simulink model "Microgrid_transition_model_092221"  (R2020a)
settings: Solver=VariableStepAuto  StartTime=0.0  StopTime=16  MaxStep=1e-4  RelTol=1e-3
PreLoadFcn:
  | %run('FC_microgrid_param.m')
  | %load('gen_grid_init.mat')
InitFcn:
  | %load myisoModel_init;
  | run('FC_microgrid_param.m')
  | tic
  | run('CARTinitFcn.m')
  | %caseNo = 2;
  | 
  | %if (caseNo == 1)
  | %set_param(['Isolated_grid_paper_model_022521/SignalGen'], 'ActiveScenario', 'PStep222kW');
  | %else
  | %set_param(['Isolated_grid_paper_model_022521/SignalGen'], 'ActiveScenario', 'QStep222kVAr');
  | 
  | %end;
StopFcn:
  | toc
undefined symbols (not defined in the file): breakpoints1, breakpoints2, cp_table_data, ctrl, D1, Delta, DiscIntNeverNeededParam, DT, FC_BESS, find_system, gcbh, libFC_BESS, LowerLimit, magnitude, oversize, pq_ts, sps_rtmsupport, timer, ts, Ts, Ts_APC, Ts_Control, Ts_Power, UpperLimit
libraries: powerlib x120, powerlib_meascontrol x85, simulink x63, powerlib_extras x40, simulink_extras x12, eePowerMeasurement x9, sps_avr x7, pi_ctrl x4, spsDieselMotorModel x3, SignalEditorBlockLib x2, libLgBattery x1, libFC_PV x1
(part 3 of 11)

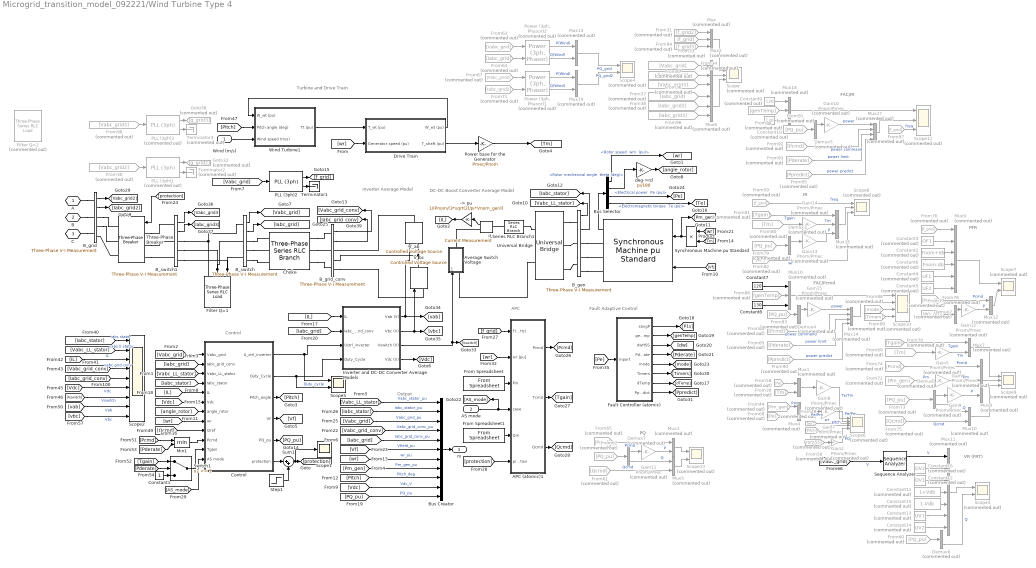
== system Microgrid_transition_model_092221/Wind Turbine Type 4 ==
  note: Control
  note: Turbine and Drive Train
  note: Inverter
      | Average Model
  note: DC-DC Boost Converter
      | Average Model
  note: Fault Adaptive Control
  note: PFR
  note: IR
  note: FAC/Pcmd
  note: PQ
  note: FAC/IR
  note: APC
  note: Output
  note: VR (FRT)
  "Wind (m/s) " : Inport
  AS mode : Inport  Port=2
  -> pu : Gain  Gain=1/(Pnom/(3*sqrt(2)/pi*Vnom_gen))  SaturateOnIntegerOverflow=on  OutDataTypeStr=Inherit: Same as input  ParamDataTypeStr=Inherit: Same as input
  APC (atomic)1 : Subsystem  TreatAsAtomicUnit=on  SystemSampleTime=0.01
  Average Switch Voltage : Subsystem
  B_gen : powerlib/Measurements/Three-Phase V-I Measurement  VoltageMeasurement=phase-to-phase  SetLabelV=off  LabelV=Vabc  Vpu=on  VpuLL=off  CurrentMeasurement=yes  SetLabelI=off  LabelI=Iabc  Ipu=on  Pbase=Pnom  Vbase=Vnom_gen  OutputType=Complex  PhasorSimulation=off  PSBequivalent=0
      settings: SourceProductBaseCode=MT,PS
  B_grid : powerlib/Measurements/Three-Phase V-I Measurement  VoltageMeasurement=phase-to-ground  SetLabelV=off  LabelV=Vabc  Vpu=off  VpuLL=off  CurrentMeasurement=yes  SetLabelI=off  LabelI=Iabc  Ipu=off  Pbase=Pnom  Vbase=Vnom  OutputType=Complex  PhasorSimulation=off  PSBequivalent=0
      settings: SourceProductBaseCode=MT,PS
  B_grid_conv : powerlib/Measurements/Three-Phase V-I Measurement  VoltageMeasurement=phase-to-ground  SetLabelV=off  LabelV=Vabc  Vpu=on  VpuLL=off  CurrentMeasurement=yes  SetLabelI=off  LabelI=Iabc  Ipu=on  Pbase=Pnom  Vbase=Vnom  OutputType=Complex  PhasorSimulation=off  PSBequivalent=0
      settings: SourceProductBaseCode=MT,PS
  B_switch : powerlib/Measurements/Three-Phase V-I Measurement  VoltageMeasurement=phase-to-ground  SetLabelV=off  LabelV=Vabc  Vpu=on  VpuLL=off  CurrentMeasurement=yes  SetLabelI=off  LabelI=Iabc  Ipu=on  Pbase=Pnom  Vbase=Vnom  OutputType=Complex  PhasorSimulation=off  PSBequivalent=0
      settings: SourceProductBaseCode=MT,PS
  B_switch1 : powerlib/Measurements/Three-Phase V-I Measurement  VoltageMeasurement=phase-to-ground  SetLabelV=off  LabelV=Vabc  Vpu=on  VpuLL=off  CurrentMeasurement=yes  SetLabelI=off  LabelI=Iabc  Ipu=on  Pbase=Pnom  Vbase=Vnom  OutputType=Complex  PhasorSimulation=off  PSBequivalent=0
      settings: SourceProductBaseCode=MT,PS
  Bus Creator : BusCreator  Inputs=11
  Bus Selector : BusSelector  OutputSignals="Mechanical.Rotor speed  wm  (pu),Mechanical.Rotor mechanical angle  theta (deg),Mechanical.Electrical power  Pe (pu),Mechanical.Electromagnetic torque  Te (pu)"
  "Choke " : powerlib/Elements/Three-Phase Series RLC Branch  LConnTagsString=A|B|C  RConnTagsString=A|B|C  BranchType=RL  Resistance=R_RL*Vnom^2/Pnom  Inductance=L_RL*Vnom^2/Pnom/(2*pi*Fnom)  Capacitance=[]  Measurements=None
      settings: SourceProductBaseCode=MT,PS
  Constant1 : Constant
  Constant10 : Constant  Commented=on  Value=130
  Constant11 : Constant  Commented=on  Value=1+Vdb
  Constant12 : Constant  Commented=on  Value=OV1
  Constant13 : Constant  Commented=on  Value=UV1
  Constant14 : Constant  Commented=on  Value=UV2
  Constant15 : Constant  Commented=on  Value=1-Vdb
  Constant16 : Constant  Commented=on  Value=OV2
  Constant2 : Constant  Commented=on  Value=Fnom+db
  Constant3 : Constant  Commented=on  Value=OF1
  Constant4 : Constant  Commented=on  Value=UF1
  Constant5 : Constant  Commented=on  Value=UF2
  Constant6 : Constant  Commented=on  Value=Fnom-db
  Constant7 : Constant  Value=120
  Constant8 : Constant  Value=130
  Constant9 : Constant  Commented=on  Value=120
  Control : Subsystem
  Demux{1..7} (7 alike) : Demux  Commented=on  Outputs=2
  Drive Train : Subsystem  mask(Wind Turbine shaft){H_WT=H_WT/10, Ksh=Ksh, D_mutual=D_mutual, wbase=2*pi*Fnom/p, w_wt0=w_wt0, torque0=torque0, Ts=Ts}
      mask prompts: H_WT "Wind turbine inertia constant H (s):"; Ksh "Shaft spring constant (pu of nominal mechanical torque/rad):"; D_mutual "Shaft mutual damping (pu of nominal mechanical torque/pu dw):"; wbase "Shaft base speed (rad/s):"; w_wt0 "Turbine initial speed (pu of base speed):"; torque0 "Initial output torque (pu of nominal mechanical torque):"; Ts "Sample time (s):"
      mask help:
      | This block implements a wind turbine drive train model. All shaft parameters are referred to high-speed shaft (generator shaft).
      |
      | The first input is the wind turbine torque in per unit (pu) based on the nominal power of the turbine and the base speed of the generator. The second input is the generator speed in pu based on the base speed of the generator.
      |
      | The outputs are:
      | 1- the transmitted torque of the shaft in pu based on the nominal power of the turbine and the base speed of the generator.
      | 2- the wind turbine speed in pu of the base speed of the generator.
  "Fault Controller (atomic) " : Subsystem  TreatAsAtomicUnit=on  SystemSampleTime=Ts_APC
  Filter Q=1 : powerlib/Elements/Three-Phase Series RLC Load  LConnTagsString=A|B|C  Configuration=Y (grounded)  NominalVoltage=Vnom  Vabc=[1e3 1e3 1e3]  Vabcp=[1e3 1e3 1e3]  NominalFrequency=Fnom  UnbalancedPower=off  ActivePower=100  InductivePower=100  CapacitivePower=100  Pabc=[10e3 9e3 11e3]  QLabc=[100 90 110]  QCabc=[100 90 110]  Pabcp=[10e3 9e3 11e3]  QLabcp=[100 90 110]  QCabcp=[100 90 110]  Measurements=None  LoadType=constant Z
      settings: SourceProductBaseCode=MT,PS
  Filter Q=2 : powerlib/Elements/Three-Phase Series RLC Load  Commented=on  LConnTagsString=A|B|C  Configuration=Y (grounded)  NominalVoltage=Vnom  Vabc=[1e3 1e3 1e3]  Vabcp=[1e3 1e3 1e3]  NominalFrequency=Fnom  UnbalancedPower=off  ActivePower=C_var_filter/Q_filter  InductivePower=0  CapacitivePower=C_var_filter  Pabc=[10e3 9e3 11e3]  QLabc=[100 90 110]  QCabc=[100 90 110]  Pabcp=[10e3 9e3 11e3]  QLabcp=[100 90 110]  QCabcp=[100 90 110]  Measurements=None  LoadType=constant Z
      settings: SourceProductBaseCode=MT,PS
  From Spreadsheet : FromSpreadsheet  FileName=Microgrid_cmd.xlsx  SheetName=P  SampleTime=Ts_APC
  From Spreadsheet1 : FromSpreadsheet  FileName=Microgrid_cmd.xlsx  SheetName=Q  SampleTime=Ts_APC
  From30 : From  Commented=on  GotoTag=Vabc_grid2
  From31 : From  Commented=on  GotoTag=f_grid2
  From{33,59,76,97} (4 alike) : From  Commented=on  GotoTag=f_grid
  From34 : From  Commented=on  GotoTag=Vabc_grid
  From36 : From  Commented=on  GotoTag=Vabc_grid2
  From37 : From  Commented=on  GotoTag=Iabc_grid
  From38 : From  Commented=on  GotoTag=Iabc_grid2
  From39 : From  Commented=on  GotoTag=Tm
  From44 : From  Commented=on  GotoTag=Pm_gen
  From48 : From  Commented=on  GotoTag=wr
  From55 : From  Commented=on  GotoTag=Pitch
  From{56,60,62,73,77,79,83,91} (8 alike) : From  Commented=on  GotoTag=PQ_pu
  From58 : From  Commented=on  GotoTag=Te
  From61 : From  Commented=on  GotoTag=Qcmd
  From63 : From  Commented=on  GotoTag=Vabc_grid
  From64 : From  Commented=on  GotoTag=Iabc_grid
  From{65,74,78,84,92} (5 alike) : From  Commented=on  GotoTag=Pcmd
  From67 : From  Commented=on  GotoTag=Vabc_grid2
  From68 : From  Commented=on  GotoTag=Pe
  From69 : From  Commented=on  GotoTag=Tm
  From70 : From  Commented=on  GotoTag=Tgain
  From71 : From  Commented=on  GotoTag=Iabc_grid2
  From72 : From  Commented=on  GotoTag=Pm_gen
  From75 : From  Commented=on  GotoTag=Qcmd
  From80 : From  Commented=on  GotoTag=Tm
  From81 : From  Commented=on  GotoTag=Tgain
  From82 : From  Commented=on  GotoTag=wr
  From85 : From  Commented=on  GotoTag=Pderate
  From86 : From  Commented=on  GotoTag=genTemp
  From87 : From  Commented=on  GotoTag=Vabc_grid3
  From88 : From  Commented=on  GotoTag=mode
  From89 : From  Commented=on  GotoTag=Timers
  From90 : From  Commented=on  GotoTag=Ppredict
  From93 : From  Commented=on  GotoTag=Pderate
  From94 : From  Commented=on  GotoTag=genTemp
  From95 : From  Commented=on  GotoTag=Ppredict
  From96 : From  Commented=on  GotoTag=Iabc_grid3
  From98 : From  Commented=on  GotoTag=Vabc_grid3
  From99 : From  Commented=on  GotoTag=f_grid3
  Gain{2,5..15} (12 alike) : Gain  Commented=on  Gain=Pnom/Pmec
  Goto32 : Goto  Commented=on  GotoTag=g_grid2
  Goto38 : Goto  Commented=on  GotoTag=g_grid3
  IL : powerlib/Measurements/Current Measurement  PhasorSimulation=off  OutputType=Complex  PSBequivalent=0
      settings: SourceProductBaseCode=MT,PS
  Inverter and DC-DC Converter Average Models : Subsystem
  Min1 : MinMax  Inputs=2
  Mux{,2,6,8,15..16,18} (7 alike) : Mux  Commented=on  Inputs=3
  Mux{1,3..5,7,10,12..13,19} (9 alike) : Mux  Commented=on  Inputs=2
  Mux11 : Mux  Commented=on  Inputs=7
  Mux14 : Mux  Commented=on
  Mux17 : Mux  Commented=on
  Mux9 : Mux  Commented=on  Inputs=6
  PLL (3ph)1 : powerlib_meascontrol/PLL/PLL (3ph)  Commented=on  Fmin=45  Par_Init=[0, 60]  ParK=[180, 3200, 1]  TcD=1e-4  MaxRateChangeFreq=12  FilterCutOffFreq=25  Ts=Ts  AGC=on
  PLL (3ph)2 : powerlib_meascontrol/PLL/PLL (3ph)  Fmin=45  Par_Init=[0, 60]  ParK=[180, 3200, 1]  TcD=1e-4  MaxRateChangeFreq=12  FilterCutOffFreq=25  Ts=Ts  AGC=on
  PLL (3ph)3 : powerlib_meascontrol/PLL/PLL (3ph)  Commented=on  Fmin=45  Par_Init=[0, 60]  ParK=[180, 3200, 1]  TcD=1e-4  MaxRateChangeFreq=12  FilterCutOffFreq=25  Ts=Ts  AGC=on
  "Power (3ph, Phasor)1" : powerlib_meascontrol/Measurements/Power (3ph, Phasor)  Commented=on
      settings: SourceProductBaseCode=PS
  "Power (3ph, Phasor)2" : powerlib_meascontrol/Measurements/Power (3ph, Phasor)  Commented=on
      settings: SourceProductBaseCode=PS
  Power base for the Generator : Gain  Gain=Pmec/Pnom  SaturateOnIntegerOverflow=on  OutDataTypeStr=Inherit: Same as input  ParamDataTypeStr=Inherit: Same as input
  Product : Product  RndMeth=Zero
  Scope{,8..9,11} (4 alike) : Scope  Commented=on  NumInputPorts=3
  Scope1 : Scope
  Scope10 : Scope  Commented=on  NumInputPorts=4
  Scope{3..4,7,13} (4 alike) : Scope  Commented=on  NumInputPorts=2
  Scope2 : Scope  NumInputPorts=9
  Scope5 : Scope  NumInputPorts=2
  Scope6 : Scope  Commented=on  NumInputPorts=5
  Sequence Analyzer : powerlib_meascontrol/Measurements/Sequence Analyzer  Freq=60  n=1  seq=Positive  InInit=[1, 0]  Ts=Ts
      settings: SourceProductBaseCode=PS
  Series RLC Branch1 : powerlib/Elements/Series RLC Branch  LConnTagsString=__new0  RConnTagsString=__new0  BranchType=RL  Resistance=R_Boost  Inductance=L_Boost  SetiL0=off  InitialCurrent=0  Capacitance=1.0  Setx0=off  InitialVoltage=0  Measurements=Branch current
      settings: SourceProductBaseCode=MT,PS
  Step1 : Step  Time=4  After=0  SampleTime=Ts
  Sum1 : Sum  Inputs=|++
  Switch1 : Switch  Threshold=1
  Synchronous Machine pu Standard : powerlib/Machines/Synchronous Machine pu Standard  PresetModel=No  MechanicalLoad=Mechanical power Pm  ShowDetailedParameters=on  RotorType=Salient-pole  Units=per unit standard parameters  MeasurementBus=off  NominalParameters="[ Pnom  Vnom_gen Fnom ]"  Reactances1=[ 1.81, 0.3, 0.23, 1.76, 0.65, 0.25, 0.15 ]  Reactances2="[ Xd, Xd1, Xd2, Xq,  Xq2,  Xl ]"  dAxisTimeConstants=Open-circuit  qAxisTimeConstants=Short-circuit  TimeConstants1="[ 4.4849  0.0681  0.1  ]"  TimeConstants2=[ 8.0, 0.03, 1.0, 0.07 ]  TimeConstants3="[  Tdo1  Tdo2  Tq2  ]"  TimeConstants4=[ 8.0, 0.03, 0.3371, 0.0295 ]  TimeConstants5=[ 1.01, 0.053, 0.1 ]  TimeConstants6=[ 1.3201, 0.023, 1.0, 0.07 ]  TimeConstants7="[  1.01  0.053  0.051266  ]"  TimeConstants8=[ 1.3201, 0.0231, 0.3371, 0.0295 ]  StatorResistance=Resistance  Mechanical=[ H F p]  PolePairs=1  InitialConditions=init  SetSaturation=off  Saturation=[0.6404,0.7127,0.8441,0.9214,0.9956,1.082,1.19,1.316,1.457;0.7,0.7698,0.8872,0.9466,0.9969,1.046,1.1,1.151,1.201]  LoadFlowParameters=[1,0,0,0,0]  TsPowergui=0  TsBlock=-1  IterativeModel=Trapezoidal non iterative  IterativeDiscreteModel=Trapezoidal non iterative  BusType=PV  Pref=0  Qref=0  Qmin=-inf  Qmax=inf  PLF=0  QLF=0
      settings: SourceProductBaseCode=MT,PS
  Terminator1 : Terminator
  Terminator2 : Terminator  Commented=on
  Terminator3 : Terminator  Commented=on
  Three-Phase Breaker : powerlib/Elements/Three-Phase Breaker  InitialState=closed  SwitchA=on  SwitchB=on  SwitchC=on  SwitchTimes=[1000]  External=on  BreakerResistance=Ron_breaker/Nb_WT  SnubberResistance=Rs_breaker/Nb_WT  SnubberCapacitance=Cs_breaker*Nb_WT  Measurements=None
  Universal Bridge : powerlib/Power Electronics/Universal Bridge  Arms=3  SnubberResistance=2*Ts_snub/(Pnom/(1000*2*pi*Fnom*Vnom_gen^2))  SnubberCapacitance=Pnom/(1000*2*pi*Fnom*Vnom_gen^2)  Device=Diodes  Ron=1e-6/Nb_wt  Lon=0  ForwardVoltages="[  0  0  ]"  ForwardVoltage=0  GTOparameters=[ 10e-6 , 20e-6 ]  IGBTparameters=[ 1e-6 , 2e-6 ]  Measurements=None  Measurements_2=None  converterType=Rectifier
      settings: SourceProductBaseCode=MT,PS
  V_ab : powerlib/Electrical Sources/Controlled Voltage Source  Initialize=on  Source_Type=AC  Amplitude=0  Phase=0  Frequency=0  Measurements=None
      settings: SourceProductBaseCode=MT,PS
  V_bc : powerlib/Electrical Sources/Controlled Voltage Source  Initialize=on  Source_Type=AC  Amplitude=0  Phase=0  Frequency=0  Measurements=None
      settings: SourceProductBaseCode=MT,PS
  Wind Turbine1 : Subsystem  mask(Wind Turbine){Prated=Pmec, c1_c8=c1_c8, K1_K2=K1_K2, wind0=wind0, Ts=Ts}
      mask prompts: Prated "Nominal mechanical output power (W):"; c1_c8 "Coefficients [c1 ... c8]"; K1_K2 "Parameters [K1 K2]"; wind0 "Initial wind speed (m/s):"; Ts "Sample time (s):"
      mask help:
      | This block implements a generic wind turbine models.
      |
      | The first input is the turbine speed in per unit of the generator base speed. For a synchronous or asynchronous generator, the base speed is the synchronous speed. For a permanent-magnet generator, the base speed is defined as the speed producing nominal voltage at  no load. The second input is the blade pitch angle in degrees. The third input is the wind speed in m/s.
      |
      | The output is the torque applied to the drive train in per unit based on the nominal power of the turbine and the base speed of the generator.
      mask init:
      | c1 = c1_c8(1);
      | c2 = c1_c8(2);
      | c3 = c1_c8(3);
      | c4 = c1_c8(4);
      | c5 = c1_c8(5);
      | c6 = c1_c8(6);
      | c7 = c1_c8(7);;
      | c8 = c1_c8(8);
      | 
      | K1=K1_K2(1);
      | K2=K1_K2(2);
      settings: OpenFcn=power_openblockproxy();
      mask Display: disp('');
  deg->rd : Gain  Gain=pi/180  SaturateOnIntegerOverflow=on  OutDataTypeStr=Inherit: Same as input  ParamDataTypeStr=Inherit: Same as input
  A : PMIOPort  Tag=PMCPort  Side=Left
  B : PMIOPort  Tag=PMCPort  Port=2  Side=Left
  C : PMIOPort  Tag=PMCPort  Port=3  Side=Left
  m : Outport  VectorParamsAs1DForOutWhenUnconnected=off
  wires:
  Bus Selector/2 -> deg->rd/1  "<Rotor mechanical angle  theta (deg)>"
  deg->rd/1 -> [angle_rotor]
  Bus Selector/1 -> [wr]  "<Rotor speed  wm  (pu)>"
  [Iabc_grid] -> Inverter and DC-DC Converter Average Models/2(Iabc_grid_conv)
  [IL] -> Inverter and DC-DC Converter Average Models/1(IL)
  [Vabc_grid] -> Control/1(Vabc_grid)
  [Iabc_grid] -> Control/2(Iabc_grid_conv)
  [Vabc_LL_stator] -> Control/3(Vabc_LL_stator)
  [Iabc_stator] -> Control/4(Iabc_stator)
  [Vdc] -> Control/6(Vdc)
  [angle_rotor] -> Control/7(angle_rotor)
  [wr] -> Control/8(wr)
  Control/2(Duty_Cycle) -> Scope5/2, Inverter and DC-DC Converter Average Models/4(Duty_Cycle)  "Duty_cycle"
  Control/3(Pitch_angle) -> [Pitch]
  Control/4(Vf) -> [Vf]
  Control/5(PQ_pu) -> [PQ_pu]
  [IL] -> Control/5(IL)
  Control/1(U_ctrl_inverter) -> Scope5/1, Inverter and DC-DC Converter Average Models/3(Uctrl_inverter)
  Inverter and DC-DC Converter Average Models/4(Vdc (V)) -> [Vdc]
  [Qcmd] -> Control/9(Qref)
  [Pitch] -> Wind Turbine1/2(Pitch angle (deg))
  Drive Train/2(T_shaft (pu)) -> Power base for the Generator/1
  Drive Train/1(W_wt (pu)) -> Wind Turbine1/1(W_wt (pu))
  "Wind (m/s) "/1 -> Wind Turbine1/3(Wind speed (m/s))
  Power base for the Generator/1 -> [Tm]
  [wr] -> Drive Train/2(Generator speed (pu))
  Wind Turbine1/1(Tt (pu)) -> Drive Train/1(T_wt (pu))
  Bus Selector/4 -> [Te]  "<Electromagnetic torque  Te (pu)>"
  Bus Selector/3 -> [Pe]  "<Electrical power  Pe (pu)>"
  Inverter and DC-DC Converter Average Models/1(Vab (V)) -> V_ab/1, [vab]
  [wr] -> Product/1
  B_gen/2 -> [Iabc_stator]
  Inverter and DC-DC Converter Average Models/2(Vbc (V)) -> V_bc/1, [vbc]
  B_switch/2 -> [Iabc_grid]
  Synchronous Machine pu Standard/1 -> Bus Selector/1
  B_switch/1 -> [Vabc_grid]
  [Tm] -> Product/2
  IL/1 -> -> pu/1
  B_gen/1 -> [Vabc_LL_stator]
  [Vf] -> Synchronous Machine pu Standard/2
  Inverter and DC-DC Converter Average Models/3(Vswitch (V)) -> Average Switch Voltage/1(Vswitch), [Vswitch]
  B_grid_conv/1 -> [Vabc_grid_conv]
  Product/1 -> Synchronous Machine pu Standard/1, [Pm_gen]
  -> pu/1 -> [IL]
  Control/6(protection) -> Sum1/1
  "Fault Controller (atomic) "/1(savgP) -> [P1s]
  [Pe] -> "Fault Controller (atomic) "/1(Inport)
  "Fault Controller (atomic) "/8(Ppredict) -> [Ppredict]
  "Fault Controller (atomic) "/2(genTemp) -> [genTemp]
  "Fault Controller (atomic) "/7(dTemp) -> [dTemp]
  "Fault Controller (atomic) "/6(Timers) -> [Timers]
  "Fault Controller (atomic) "/4(Pderate) -> [Pderate]
  "Fault Controller (atomic) "/3(dwHSS) -> [dw]
  "Fault Controller (atomic) "/5(mode) -> [mode]
  Gain8/1 -> Scope6/1  "Te/Tm"
  From80/1 -> Gain14/1
  From77/1 -> Demux2/1
  From39/1 -> Mux1/2
  Constant10/1 -> Mux18/3
  From75/1 -> Mux10/2  "Qcmd"
  Mux12/1 -> Scope7/2
  From74/1 -> Mux8/1  "Pcmd"
  From58/1 -> Mux1/1
  Mux9/1 -> Scope7/1
  From83/1 -> Demux4/1
  Gain13/1 -> Mux15/3  "P"
  Gain14/1 -> Mux15/2  "Tm"
  Gain12/1 -> Mux12/2  "P"
  From70/1 -> Mux7/1  "Tgain"
  Demux5/1 -> Gain10/1
  Gain9/1 -> Mux8/3  "P"
  From85/1 -> Mux14/3  "power limit"
  From68/1 -> Mux4/2
  From82/1 -> Scope8/3  "wr"
  Mux17/1 -> Scope11/2
  Demux1/1 -> Gain9/1
  From89/1 -> Scope10/4
  Mux5/1 -> Scope13/2
  Mux4/1 -> Gain7/1  "Pe/Pm"
  From59/1 -> Scope8/1  "freq"
  From90/1 -> Mux14/4  "power predict"
  Mux10/1 -> Scope9/3
  Demux1/2 -> Mux10/1  "Q"
  From44/1 -> Mux4/1  "Pm"
  From94/1 -> Mux18/2
  From55/1 -> Scope6/4  "pitch"
  Mux14/1 -> Scope10/2
  From56/1 -> Gain2/1
  Constant9/1 -> Mux18/1
  Constant8/1 -> Mux16/3
  From73/1 -> Demux1/1
  From93/1 -> Mux17/3  "power limit"
  From92/1 -> Mux17/2  "power command"
  Mux1/1 -> Gain8/1
  Mux8/1 -> Scope9/2
  Gain15/1 -> Mux14/1  "power"
  Constant2/1 -> Mux9/3
  Mux16/1 -> Scope10/1
  From84/1 -> Mux14/2  "power command"
  From78/1 -> Mux12/1  "Pcmd"
  Constant7/1 -> Mux16/1
  Mux15/1 -> Scope8/2
  From91/1 -> Demux5/1
  Gain11/1 -> Mux3/2  "P"
  Gain5/1 -> Mux7/2  "Tm"
  From72/1 -> Gain6/1  "Pm"
  From62/1 -> Demux7/1
  From97/1 -> Scope11/3  "freq"
  Gain10/1 -> Mux17/1  "power"
  From81/1 -> Mux15/1  "Tgain"
  Gain6/1 -> Mux8/2  "Pm"
  From61/1 -> Mux5/2  "Qcmd"
  From69/1 -> Gain5/1
  From48/1 -> Scope6/3  "wr"
  Mux3/1 -> Scope13/1
  Demux2/1 -> Gain12/1
  Demux4/1 -> Gain15/1
  Constant3/1 -> Mux9/2
  Constant5/1 -> Mux9/6
  Demux7/2 -> Mux5/1  "Q"
  From79/1 -> Demux3/1
  From65/1 -> Mux3/1  "Pcmd"
  From95/1 -> Mux17/4  "power predict"
  Constant6/1 -> Mux9/4
  Demux3/1 -> Gain13/1
  Constant4/1 -> Mux9/5
  Gain2/1 -> Scope6/5  "PQ"
  Demux7/1 -> Gain11/1
  Mux18/1 -> Scope11/1
  Mux7/1 -> Scope9/1
  From76/1 -> Mux9/1
  Gain7/1 -> Scope6/2  "Pe/Pm"
  From88/1 -> Scope10/3
  From86/1 -> Mux16/2
  [Pderate] -> Min1/2
  [Pcmd] -> Min1/1
  Min1/1 -> Control/10(Pcmd)
  [Pderate] -> Switch1/2
  Switch1/1 -> Control/11(Tgain)
  Constant1/1 -> Switch1/3
  [Tgain] -> Switch1/1
  PLL (3ph)2/2 -> Terminator1/1
  [Vabc_grid] -> PLL (3ph)2/1
  PLL (3ph)2/1 -> [f_grid]
  From Spreadsheet1/1 -> APC (atomic)1/5(Qin)
  [f_grid] -> APC (atomic)1/1(Freq (Hz))
  APC (atomic)1/3(Qcmd) -> [Qcmd]
  APC (atomic)1/2(Tcmd) -> [Tgain]
  [protection] -> APC (atomic)1/6(protection)
  [wr] -> APC (atomic)1/2(wr [pu])
  AS mode/1 -> APC (atomic)1/4(case), [AS_mode]
  APC (atomic)1/1(Pcmd) -> [Pcmd]
  From Spreadsheet/1 -> APC (atomic)1/3(Pin)
  [AS_mode] -> Control/12(AS mode)
  [Pm_gen] -> Bus Creator/8  "Pm_gen_pu"
  Bus Creator/1 -> m/1
  [Iabc_grid] -> Bus Creator/5  "Iabc_grid_conv_pu"
  [Pitch] -> Bus Creator/9  "Pitch_deg"
  [PQ_pu] -> Bus Creator/11  "PQ_pu"
  [Vf] -> Bus Creator/6  "Vfield_pu"
  [Vdc] -> Bus Creator/10  "Vdc_V"
  [Vabc_LL_stator] -> Bus Creator/1  "Vabc_stator_pu"
  [Vabc_grid] -> Bus Creator/3  "Vabc_grid_pu"
  [Iabc_stator] -> Bus Creator/2  "Iabc_stator_pu"
  [wr] -> Bus Creator/7  "wr_pu"
  [Vabc_grid_conv] -> Bus Creator/4  "Vabc_grid_conv_pu"
  B_grid/2 -> [Iabc_grid2]
  B_grid/1 -> [Vabc_grid2]
  PLL (3ph)1/1 -> Goto32/1
  PLL (3ph)1/2 -> Terminator2/1
  From30/1 -> PLL (3ph)1/1
  From31/1 -> Mux/1
  From33/1 -> Mux/2
  From34/1 -> Mux2/1
  From36/1 -> Mux2/2
  Mux2/1 -> Scope/2
  Mux/1 -> Scope/1
  [protection] -> Three-Phase Breaker/1
  Step1/1 -> Sum1/2
  Sum1/1 -> Scope1/1, [protection]
  [Iabc_stator] -> Scope2/1  "iabc stator"
  [Vabc_LL_stator] -> Scope2/2  "vabs ll stator"
  [IL] -> Scope2/3  "IL"
  [Vabc_grid_conv] -> Scope2/4  "vabc grid conv"
  [Vdc] -> Scope2/6  "Vdc"
  [Vswitch] -> Scope2/7  "Vswitch"
  [vab] -> Scope2/8  "Vab"
  [vbc] -> Scope2/9  "Vbc"
  Sequence Analyzer/1 -> Mux11/1  "V"
  Constant13/1 -> Mux11/6
  Constant15/1 -> Mux11/5
  Constant14/1 -> Mux11/7
  Constant12/1 -> Mux11/3
  Constant11/1 -> Mux11/4
  Mux11/1 -> Scope3/1
  [Vabc_grid] -> Sequence Analyzer/1  "V"
  Constant16/1 -> Mux11/2
  Demux6/2 -> Scope3/2  "Q"
  From60/1 -> Demux6/1
  "Power (3ph, Phasor)2"/2 -> Mux13/2  "Q(Wind)"
  From63/1 -> "Power (3ph, Phasor)2"/1
  "Power (3ph, Phasor)2"/1 -> Mux13/1  "P(Wind)"
  From64/1 -> "Power (3ph, Phasor)2"/2
  Mux13/1 -> Scope4/1  "PQ_grid"
  Mux19/1 -> Scope4/2  "PQ_grid2"
  From71/1 -> "Power (3ph, Phasor)1"/2
  From67/1 -> "Power (3ph, Phasor)1"/1
  "Power (3ph, Phasor)1"/1 -> Mux19/1  "P(Wind)"
  "Power (3ph, Phasor)1"/2 -> Mux19/2  "Q(Wind)"
  B_switch1/1 -> [Vabc_grid3]
  B_switch1/2 -> [Iabc_grid3]
  PLL (3ph)3/1 -> Goto38/1
  PLL (3ph)3/2 -> Terminator3/1
  From98/1 -> PLL (3ph)3/1
  From99/1 -> Mux/3
  From87/1 -> Mux2/3
  From37/1 -> Mux6/1
  From38/1 -> Mux6/2
  From96/1 -> Mux6/3
  Mux6/1 -> Scope/3
  B_grid_conv/2 -> [Iabc_grid_conv]
  [Iabc_grid_conv] -> Scope2/5
  connections:
  B_grid/RConn1 -- Three-Phase Breaker/RConn1
  B_grid/RConn2 -- Three-Phase Breaker/RConn2
  Three-Phase Breaker/RConn3 -- B_grid/RConn3
  B_grid_conv/RConn2 -- V_bc/RConn1 -- V_ab/LConn1
  Filter Q=1/LConn3 -- B_switch/LConn3 -- B_switch1/RConn3
  Filter Q=1/LConn2 -- B_switch/LConn2 -- B_switch1/RConn2
  B_switch/LConn1 -- B_switch1/RConn1 -- Filter Q=1/LConn1
  B_switch/RConn3 -- "Choke "/LConn3
  "Choke "/RConn3 -- B_grid_conv/LConn3
  B_switch/RConn2 -- "Choke "/LConn2
  Universal Bridge/LConn1 -- B_gen/LConn1
  B_gen/RConn2 -- Synchronous Machine pu Standard/RConn2
  Average Switch Voltage/RConn1 -- IL/RConn1
  Universal Bridge/LConn2 -- B_gen/LConn2
  Universal Bridge/LConn3 -- B_gen/LConn3
  V_ab/RConn1 -- B_grid_conv/RConn1
  B_switch/RConn1 -- "Choke "/LConn1
  B_gen/RConn1 -- Synchronous Machine pu Standard/RConn1
  "Choke "/RConn1 -- B_grid_conv/LConn1
  "Choke "/RConn2 -- B_grid_conv/LConn2
  B_grid_conv/RConn3 -- V_bc/LConn1
  Series RLC Branch1/LConn1 -- Universal Bridge/RConn1
  B_gen/RConn3 -- Synchronous Machine pu Standard/RConn3
  Series RLC Branch1/RConn1 -- IL/LConn1
  Average Switch Voltage/LConn1 -- Universal Bridge/RConn2
  A/RConn1 -- B_grid/LConn1
  B/RConn1 -- B_grid/LConn2
  C/RConn1 -- B_grid/LConn3
  Three-Phase Breaker/LConn1 -- B_switch1/LConn1
  Three-Phase Breaker/LConn2 -- B_switch1/LConn2
  Three-Phase Breaker/LConn3 -- B_switch1/LConn3

== system Microgrid_transition_model_092221/induction attempts2 ==
  Asynchronous Machine pu ABB 1.8MW : powerlib/Machines/Asynchronous Machine pu Units  Commented=on  RotorType=Squirrel-cage  PresetModel=No  MechanicalLoad=Torque Tm  ShowDetailedParameters=on  ReferenceFrame=Rotor  Units=pu  MeasurementBus=off  NominalParameters=[1.8e+06 1e+04 60]  Stator=[0.02565 0.09937]  Rotor=[0.01909 0.0397]  Cage1=[0.004672 0.11]  Cage2=[0.04455 0.09937]  Lm=3.275  Mechanical=[0.09526 0.05479 2]  PolePairs=2  InitialConditions="[ 0.01,0   0,0,0   0,0,0 ]"  SimulateSaturation=off  Saturation="[0.212,0.4201,0.8125,1.0979,1.4799,2.2457,3.2586,4.5763,6.4763 ;   0.5,0.7,0.9,1,1.1,1.2 ,1.3,1.4,1.5]"  LoadFlowParameters=0  TsPowergui=0  TsBlock=-1  IterativeModel=Trapezoidal non iterative  IterativeDiscreteModel=Trapezoidal non iterative  Pmec=0
      settings: SourceProductBaseCode=PS
  Asynchronous Machine pu Baldor 500HP : powerlib/Machines/Asynchronous Machine pu Units  RotorType=Squirrel-cage  PresetModel=No  MechanicalLoad=Torque Tm  ShowDetailedParameters=on  ReferenceFrame=Rotor  Units=pu  MeasurementBus=off  NominalParameters=[3.731e+05 460 60]  Stator=[0.02671 0.07843]  Rotor=[0.01909 0.0397]  Cage1=[0.00673 0.1222]  Cage2=[0.05602 0.07843]  Lm=3.861  Mechanical=[0.09526 0.05479 1]  PolePairs=2  InitialConditions="[ 0.01,0   0,0,0   0,0,0 ]"  SimulateSaturation=off  Saturation="[0.212,0.4201,0.8125,1.0979,1.4799,2.2457,3.2586,4.5763,6.4763 ;   0.5,0.7,0.9,1,1.1,1.2 ,1.3,1.4,1.5]"  LoadFlowParameters=0  TsPowergui=0  TsBlock=-1  IterativeModel=Trapezoidal non iterative  IterativeDiscreteModel=Trapezoidal non iterative  Pmec=0
      settings: SourceProductBaseCode=PS
  Asynchronous Machine pu FCgen : powerlib/Machines/Asynchronous Machine pu Units  Commented=on  RotorType=Squirrel-cage  PresetModel=No  MechanicalLoad=Torque Tm  ShowDetailedParameters=on  ReferenceFrame=Rotor  Units=pu  MeasurementBus=off  NominalParameters=[2.02e+06 460 60]  Stator=[-0.005 0.09337]  Rotor=[0.01909 0.0397]  Cage1=[-0.01 0.2054]  Cage2=[-0.06 0.09337]  Lm=1.867  Mechanical=[0.09526 0.05479 1]  PolePairs=2  InitialConditions="[ 0.01, 0,   0,0,0   0,0,0 ]"  SimulateSaturation=off  Saturation="[0.212,0.4201,0.8125,1.0979,1.4799,2.2457,3.2586,4.5763,6.4763 ;   0.5,0.7,0.9,1,1.1,1.2 ,1.3,1.4,1.5]"  LoadFlowParameters=0  TsPowergui=0  TsBlock=Ts  IterativeModel=Trapezoidal non iterative  IterativeDiscreteModel=Trapezoidal non iterative  Pmec=0
      settings: SourceProductBaseCode=PS
  Bus Selector : BusSelector  OutputSignals=Mechanical.Electromagnetic torque Te (pu),Mechanical.Rotor speed (wm)
  Bus Selector2 : BusSelector  OutputSignals=Mechanical.Rotor speed (wm)  OutputAsBus=on
  Diesel Engine Governor : spsDieselMotorModel/Diesel Engine Governor  K=10/4  Tr=[0.01 0.02 0.2]  Ta=[0.2 0.009 0.0384]  Tlim=[0 1.1]  Td=0.05  Pm0=0.126/0.126
      settings: SourceProductBaseCode=PS
  Divide : Product  Inputs=*/
  Divide1 : Product  Inputs=**
  Gain1 : Gain  Gain=1.8e6
  SM 3.125 MVA1 : powerlib/Machines/Synchronous Machine pu Standard  Commented=on  PresetModel=No  MechanicalLoad=Mechanical power Pm  ShowDetailedParameters=on  RotorType=Salient-pole  Units=per unit standard parameters  MeasurementBus=off  NominalParameters=[2e+06 460 60]  Reactances1=[ 31 32 33 34 35 36 37 ]  Reactances2=[3.08 0.24 0.18 2.28 0.23 0.04]  dAxisTimeConstants=Short-circuit  qAxisTimeConstants=Short-circuit  TimeConstants1=[]  TimeConstants2=[]  TimeConstants3=[]  TimeConstants4=[]  TimeConstants5=[ 3.7, 0.05, 0.05 ]  TimeConstants6=[ 8.0, 0.03, 0.3371, 0.0295 ]  TimeConstants7=[0.29 0.03 0.03]  TimeConstants8=[]  StatorResistance=0.012007561436673  Mechanical=[1 0.01231 2]  PolePairs=2  InitialConditions=[0 0 0 0 0 0 0 0 1]  SetSaturation=off  Saturation=[0.211 0.418 1.0 1.25 1.72 3.35 ;0.25 0.50 1.0 1.1 1.2 1.4]  LoadFlowParameters=[1 0 0 0]  TsPowergui=0  TsBlock=Ts  IterativeModel=Trapezoidal non iterative  IterativeDiscreteModel=Backward Euler robust  BusType=PV  Pref=0  Qref=0  Qmin=-Inf  Qmax=Inf  PLF=0  QLF=0
      settings: AttributesFormatString=\n\n  SourceProductBaseCode=MT,PS
  Scope : Scope  NumInputPorts=3
  Scope1 : Scope  NumInputPorts=3
  Scope2 : Scope
  wref (pu) : Constant
  A : PMIOPort  Side=Right
  B : PMIOPort  Port=2  Side=Right
  C : PMIOPort  Port=3  Side=Right
  wires:
  Asynchronous Machine pu Baldor 500HP/1 -> Bus Selector/1, Bus Selector2/1
  Diesel Engine Governor/1 -> Scope1/1, Divide/1  "Pm"
  wref (pu)/1 -> Diesel Engine Governor/1
  Bus Selector2/1 -> Scope1/3, Divide/2, Diesel Engine Governor/2  "Wm"
  Divide/1 -> Asynchronous Machine pu Baldor 500HP/1, Scope1/2
  Bus Selector/1 -> Scope/2, Divide1/1  "<Electromagnetic torque Te (pu)>"
  Bus Selector/2 -> Scope/1, Divide1/2  "<Rotor speed (wm)>"
  Divide1/1 -> Gain1/1, Scope/3
  Gain1/1 -> Scope2/1
  connections:
  Asynchronous Machine pu Baldor 500HP/LConn3 -- C/RConn1
  Asynchronous Machine pu Baldor 500HP/LConn1 -- A/RConn1
  Asynchronous Machine pu Baldor 500HP/LConn2 -- B/RConn1

== system Microgrid_transition_model_092221/synchronous ==
  note: try adding a delay to Vf
  Bus Selector : BusSelector  OutputSignals="Output active power   Peo (pu),Output reactive power  Qeo (pu),Mechanical.Electrical power  Pe (pu)"
  Bus Selector2 : BusSelector  OutputSignals="Mechanical.Rotor speed  wm  (pu)"  OutputAsBus=on
  Bus Selector4 : BusSelector  OutputSignals="dq0 components.Field current  ifd (pu)"  OutputAsBus=on
  Bus Selector5 : BusSelector  OutputSignals="dq0 components.Stator voltage  vd (pu),dq0 components.Stator voltage  vq (pu)"  OutputAsBus=on
  Bus Selector6 : BusSelector  OutputSignals="dq0 components.Stator current  id (pu),dq0 components.Stator current  iq (pu)"  OutputAsBus=on
  Delay : Delay  DelayLength=0
  Diesel Engine Governor : spsDieselMotorModel/Diesel Engine Governor  K=10  Tr=[0.01 0.02 0.2]  Ta=[0.2 0.009 0.0384]  Tlim=[0 1.1]  Td=0.05  Pm0=0.126
      settings: SourceProductBaseCode=PS
  EXCITATION : Subsystem  Variant=on  VariantControlMode=Label  LabelModeActiveChoice=Variant1
      settings: AttributesFormatString=%<BlockChoice>
  Fcn1 : Fcn  Expr=sqrt(u(1)^2 + u(2)^2)
  Fcn2 : Fcn  Expr=sqrt(u(1)^2 + u(2)^2)
  Ground : Ground
  SM : Scope  NumInputPorts=4
  SM 3.125 MVA : powerlib/Machines/Synchronous Machine pu Standard  PresetModel=No  MechanicalLoad=Mechanical power Pm  ShowDetailedParameters=on  RotorType=Salient-pole  Units=per unit standard parameters  MeasurementBus=off  NominalParameters=[2e+06 460 60]  Reactances1=[ 31 32 33 34 35 36 37 ]  Reactances2=[3.08 0.24 0.18 2.28 0.23 0.04]  dAxisTimeConstants=Short-circuit  qAxisTimeConstants=Short-circuit  TimeConstants1=[]  TimeConstants2=[]  TimeConstants3=[]  TimeConstants4=[]  TimeConstants5=[ 3.7, 0.05, 0.05 ]  TimeConstants6=[ 8.0, 0.03, 0.3371, 0.0295 ]  TimeConstants7=[0.29 0.03 0.03]  TimeConstants8=[]  StatorResistance=0.012007561436673  Mechanical=[1 0.01231 2]  PolePairs=2  InitialConditions=[0 0 0 0 0 0 0 0 1]  SetSaturation=off  Saturation=[0.211 0.418 1.0 1.25 1.72 3.35 ;0.25 0.50 1.0 1.1 1.2 1.4]  LoadFlowParameters=[1 0 0 0]  TsPowergui=0  TsBlock=Ts  IterativeModel=Trapezoidal non iterative  IterativeDiscreteModel=Backward Euler robust  BusType=PV  Pref=0  Qref=0  Qmin=-Inf  Qmax=Inf  PLF=0  QLF=0
      settings: AttributesFormatString=\n\n  SourceProductBaseCode=MT,PS
  Scope : Scope  NumInputPorts=3
  Scope1 : Scope
  "Vtref (pu) " : Constant
  wref (pu) : FromSpreadsheet  FileName=Microgrid_cmd.xlsx  SheetName=wref  SampleTime=Ts_APC
  A : PMIOPort  Side=Right
  B : PMIOPort  Port=2  Side=Right
  C : PMIOPort  Port=3  Side=Right
  wires:
  wref (pu)/1 -> Diesel Engine Governor/1, Scope1/1
  Bus Selector5/1 -> Fcn1/1  "Vd Vq"
  SM 3.125 MVA/1 -> Bus Selector/1, Bus Selector2/1, Bus Selector4/1, Bus Selector6/1, Bus Selector5/1
  Fcn2/1 -> EXCITATION/3(It)
  "Vtref (pu) "/1 -> EXCITATION/1(Vref)
  Bus Selector6/1 -> Fcn2/1  "Id Iq"
  EXCITATION/1(Efd) -> Delay/1  "Vf"
  Bus Selector4/1 -> EXCITATION/4(Ifd)  "Ifd"
  Diesel Engine Governor/1 -> SM 3.125 MVA/1, SM/2  "Pm"
  Ground/1 -> EXCITATION/5(Vstab)  "Not implemented"
  Fcn1/1 -> SM/4, EXCITATION/2(Vt)  "Vt"
  Bus Selector2/1 -> SM/1, Diesel Engine Governor/2  "Wm"
  Bus Selector/1 -> Scope/1  "<Output active power   Peo (pu)>"
  Bus Selector/2 -> Scope/2  "<Output reactive power  Qeo (pu)>"
  Bus Selector/3 -> Scope/3  "<Electrical power  Pe (pu)>"
  Delay/1 -> SM/3, SM 3.125 MVA/2
  connections:
  SM 3.125 MVA/RConn3 -- C/RConn1
  SM 3.125 MVA/RConn1 -- A/RConn1
  SM 3.125 MVA/RConn2 -- B/RConn1

== system Microgrid_transition_model_092221/uhhh ==
  Asynchronous Machine pu Units : powerlib/Machines/Asynchronous Machine pu Units  RotorType=Double squirrel-cage  PresetModel=No  MechanicalLoad=Torque Tm  ShowDetailedParameters=on  ReferenceFrame=Rotor  Units=pu  MeasurementBus=off  NominalParameters=[2.02e+06 460 60]  Stator=[-0.005 0.09337]  Rotor=[0.01909 0.0397]  Cage1=[-0.01 0.2054]  Cage2=[-0.06 0.09337]  Lm=1.867  Mechanical=[0.09526 0.05479 1]  PolePairs=2  InitialConditions="[ 1,0   0,0,0   0,0,0 ]"  SimulateSaturation=off  Saturation="[0.212,0.4201,0.8125,1.0979,1.4799,2.2457,3.2586,4.5763,6.4763 ;   0.5,0.7,0.9,1,1.1,1.2 ,1.3,1.4,1.5]"  LoadFlowParameters=0  TsPowergui=0  TsBlock=Ts  IterativeModel=Trapezoidal non iterative  IterativeDiscreteModel=Trapezoidal non iterative  Pmec=0
      settings: SourceProductBaseCode=PS
  Bus Selector : BusSelector  OutputSignals=Mechanical.Electromagnetic torque Te (pu),Mechanical.Rotor speed (wm)
  Bus Selector2 : BusSelector  OutputSignals=Mechanical.Rotor speed (wm)  OutputAsBus=on
  Diesel Engine Governor : spsDieselMotorModel/Diesel Engine Governor  K=10  Tr=[0.01 0.02 0.2]  Ta=[0.2 0.009 0.0384]  Tlim=[0 1.1]  Td=0.05  Pm0=0.126
      settings: SourceProductBaseCode=PS
  Divide : Product  Inputs=*/
  Divide1 : Product  Inputs=**
  Gain : Gain  Gain=2.02e6
  SM 3.125 MVA1 : powerlib/Machines/Synchronous Machine pu Standard  PresetModel=No  MechanicalLoad=Mechanical power Pm  ShowDetailedParameters=on  RotorType=Salient-pole  Units=per unit standard parameters  MeasurementBus=off  NominalParameters=[2e+06 460 60]  Reactances1=[ 31 32 33 34 35 36 37 ]  Reactances2=[3.08 0.24 0.18 2.28 0.23 0.04]  dAxisTimeConstants=Short-circuit  qAxisTimeConstants=Short-circuit  TimeConstants1=[]  TimeConstants2=[]  TimeConstants3=[]  TimeConstants4=[]  TimeConstants5=[ 3.7, 0.05, 0.05 ]  TimeConstants6=[ 8.0, 0.03, 0.3371, 0.0295 ]  TimeConstants7=[0.29 0.03 0.03]  TimeConstants8=[]  StatorResistance=0.012007561436673  Mechanical=[1 0.01231 2]  PolePairs=2  InitialConditions=[0 0 0 0 0 0 0 0 1]  SetSaturation=off  Saturation=[0.211 0.418 1.0 1.25 1.72 3.35 ;0.25 0.50 1.0 1.1 1.2 1.4]  LoadFlowParameters=[1 0 0 0]  TsPowergui=0  TsBlock=Ts  IterativeModel=Trapezoidal non iterative  IterativeDiscreteModel=Backward Euler robust  BusType=PV  Pref=0  Qref=0  Qmin=-Inf  Qmax=Inf  PLF=0  QLF=0
      settings: AttributesFormatString=\n\n  SourceProductBaseCode=MT,PS
  Scope : Scope  NumInputPorts=3
  wref (pu) : Constant
  A : PMIOPort  Side=Right
  B : PMIOPort  Port=2  Side=Right
  C : PMIOPort  Port=3  Side=Right
  wires:
  Gain/1 -> Scope/3
  Divide1/1 -> Gain/1
  Bus Selector/2 -> Divide1/2, Scope/1  "<Rotor speed (wm)>"
  Bus Selector/1 -> Divide1/1, Scope/2  "<Electromagnetic torque Te (pu)>"
  Divide/1 -> Asynchronous Machine pu Units/1
  Bus Selector2/1 -> Diesel Engine Governor/2, Divide/2  "Wm"
  wref (pu)/1 -> Diesel Engine Governor/1
  Diesel Engine Governor/1 -> Divide/1  "Pm"
  Asynchronous Machine pu Units/1 -> Bus Selector2/1, Bus Selector/1
  connections:
  B/RConn1 -- Asynchronous Machine pu Units/LConn2
  A/RConn1 -- Asynchronous Machine pu Units/LConn1
  C/RConn1 -- Asynchronous Machine pu Units/LConn3

== system Microgrid_transition_model_092221/../Average Switch Voltage ==
  Vswitch : Inport
  Diode : powerlib/Power Electronics/Diode  Ron=1e-6/Nb_wt  Lon=0  Vf=0  IC=0  UseSnubber=off  Rs=1e5  Cs=inf  Measurements=off
      settings: SourceProductBaseCode=MT,PS
  V : powerlib/Electrical Sources/Controlled Voltage Source  Initialize=on  Source_Type=AC  Amplitude=0  Phase=0  Frequency=0  Measurements=None
      settings: SourceProductBaseCode=MT,PS
  + : PMIOPort  Side=Right
  - : PMIOPort  Port=2  Side=Left
  wires:
  Vswitch/1 -> V/1
  connections:
  -/RConn1 -- V/LConn1
  +/RConn1 -- Diode/LConn1
  Diode/RConn1 -- V/RConn1

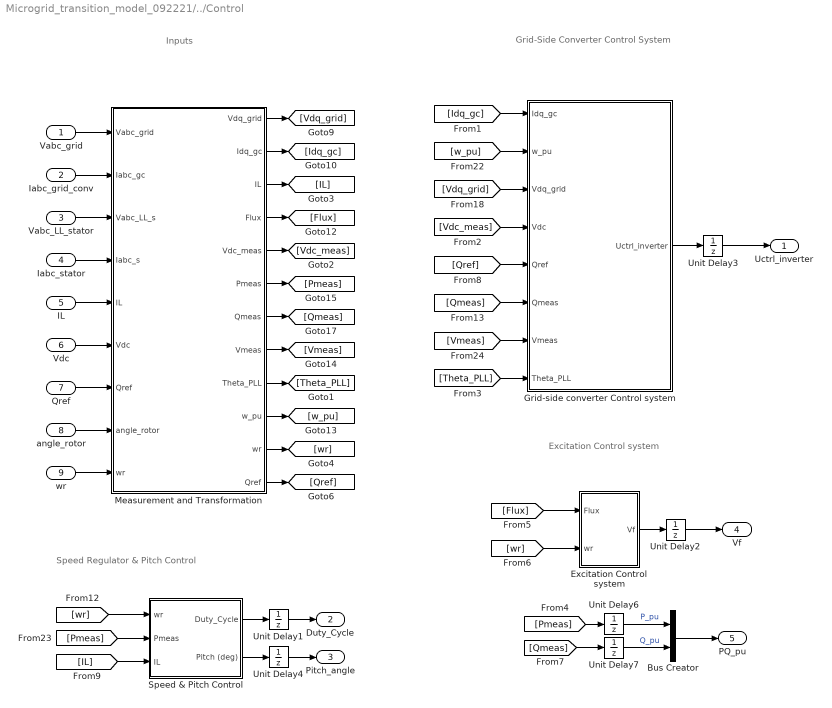
== system Microgrid_transition_model_092221/../Control ==
  note: Excitation
      | Control system
  note: Speed Regulator & Pitch Control
  note: Grid-Side Converter
      | Control System
  note: Inputs
  Vabc_grid : Inport
  Iabc_grid_conv : Inport  Port=2
  Vabc_LL_stator : Inport  Port=3
  Iabc_stator : Inport  Port=4
  IL : Inport  Port=5
  Vdc : Inport  Port=6
  Qref : Inport  Port=7
  angle_rotor : Inport  Port=8
  wr : Inport  Port=9
  Bus Creator : BusCreator  Inputs=2
  Excitation Control system : Subsystem
  Grid-side converter Control system : Subsystem
  Measurement and Transformation : Subsystem
  Speed & Pitch Control : Subsystem
  Unit Delay{1..4,6..7} (6 alike) : UnitDelay  SampleTime=Ts  HasFrameUpgradeWarning=on
  Uctrl_inverter : Outport  VectorParamsAs1DForOutWhenUnconnected=off
  Duty_Cycle : Outport  Port=2  VectorParamsAs1DForOutWhenUnconnected=off
  Pitch_angle : Outport  Port=3  VectorParamsAs1DForOutWhenUnconnected=off
  Vf : Outport  Port=4  VectorParamsAs1DForOutWhenUnconnected=off
  PQ_pu : Outport  Port=5  VectorParamsAs1DForOutWhenUnconnected=off
  wires:
  [IL] -> Speed & Pitch Control/3(IL)
  IL/1 -> Measurement and Transformation/5(IL)
  Measurement and Transformation/3("IL ") -> [IL]
  Unit Delay7/1 -> Bus Creator/2  "Q_pu"
  Unit Delay6/1 -> Bus Creator/1  "P_pu"
  [Qmeas] -> Unit Delay7/1
  [Pmeas] -> Unit Delay6/1
  Unit Delay4/1 -> Pitch_angle/1
  Unit Delay1/1 -> Duty_Cycle/1
  Unit Delay2/1 -> Vf/1
  Unit Delay3/1 -> Uctrl_inverter/1
  Bus Creator/1 -> PQ_pu/1
  Measurement and Transformation/9(Theta_PLL) -> [Theta_PLL]
  [Theta_PLL] -> Grid-side converter Control system/8(Theta_PLL)
  Grid-side converter Control system/1(Uctrl_inverter) -> Unit Delay3/1
  wr/1 -> Measurement and Transformation/9(wr)
  angle_rotor/1 -> Measurement and Transformation/8(angle_rotor)
  Qref/1 -> Measurement and Transformation/7(Qref)
  Vdc/1 -> Measurement and Transformation/6(Vdc)
  Iabc_stator/1 -> Measurement and Transformation/4(Iabc_s)
  Vabc_LL_stator/1 -> Measurement and Transformation/3(Vabc_LL_s)
  Iabc_grid_conv/1 -> Measurement and Transformation/2(Iabc_gc)
  Vabc_grid/1 -> Measurement and Transformation/1(Vabc_grid)
  [wr] -> Excitation Control system/2(wr)
  [Flux] -> Excitation Control system/1(Flux)
  Measurement and Transformation/4(Flux) -> [Flux]
  Speed & Pitch Control/1(Duty_Cycle) -> Unit Delay1/1
  [Pmeas] -> Speed & Pitch Control/2(Pmeas)
  [wr] -> Speed & Pitch Control/1(wr)
  [Vmeas] -> Grid-side converter Control system/7(Vmeas)
  [Qmeas] -> Grid-side converter Control system/6(Qmeas)
  [Qref] -> Grid-side converter Control system/5(Qref)
  Measurement and Transformation/12("Qref ") -> [Qref]
  Measurement and Transformation/11("wr ") -> [wr]
  Measurement and Transformation/5(Vdc_meas) -> [Vdc_meas]
  [Vdc_meas] -> Grid-side converter Control system/4(Vdc)
  [Vdq_grid] -> Grid-side converter Control system/3(Vdq_grid)
  [w_pu] -> Grid-side converter Control system/2(w_pu)
  [Idq_gc] -> Grid-side converter Control system/1(Idq_gc)
  Measurement and Transformation/10(w_pu) -> [w_pu]
  Measurement and Transformation/8(Vmeas) -> [Vmeas]
  Measurement and Transformation/6(Pmeas) -> [Pmeas]
  Measurement and Transformation/2(Idq_gc) -> [Idq_gc]
  Measurement and Transformation/1(Vdq_grid) -> [Vdq_grid]
  Measurement and Transformation/7(Qmeas) -> [Qmeas]
  Speed & Pitch Control/2(Pitch (deg)) -> Unit Delay4/1
  Excitation Control system/1(Vf) -> Unit Delay2/1

== system Microgrid_transition_model_092221/../Drive Train ==
  note: Shaft
  note: Turbine
  note: Wind turbine drive train based on a 2-masse model
  T_wt (pu) : Inport
  Generator speed (pu) : Inport  Port=2
  1_2H_WT : Gain  Gain=1/(2*H_WT)  SaturateOnIntegerOverflow=on  OutDataTypeStr=Inherit: Same as input  ParamDataTypeStr=Inherit: Same as input
  Discrete-Time Integrator : DiscreteIntegrator  InitialCondition=w_wt0  SampleTime=Ts  ICPrevOutput=DiscIntNeverNeededParam  ICPrevScaledInput=DiscIntNeverNeededParam
  Discrete-Time Integrator1 : DiscreteIntegrator  InitialCondition=torque0/Ksh  SampleTime=Ts  ICPrevOutput=DiscIntNeverNeededParam  ICPrevScaledInput=DiscIntNeverNeededParam
  Mutual damping : Gain  Gain=D_mutual  SaturateOnIntegerOverflow=on  OutDataTypeStr=Inherit: Same as input  ParamDataTypeStr=Inherit: Same as input
  Stiffness : Gain  Gain=Ksh  SaturateOnIntegerOverflow=on  OutDataTypeStr=Inherit: Same as input  ParamDataTypeStr=Inherit: Same as input
  Sum : Sum  Inputs=+-  InputSameDT=on  SaturateOnIntegerOverflow=on  OutDataTypeStr=Inherit: Same as first input
  Sum1 : Sum  Inputs=+-  InputSameDT=on  SaturateOnIntegerOverflow=on  OutDataTypeStr=Inherit: Same as first input
  Sum2 : Sum  InputSameDT=on  SaturateOnIntegerOverflow=on  OutDataTypeStr=Inherit: Same as first input
  wbase : Gain  Gain=wbase  SaturateOnIntegerOverflow=on  OutDataTypeStr=Inherit: Same as input  ParamDataTypeStr=Inherit: Same as input
  W_wt (pu) : Outport  VectorParamsAs1DForOutWhenUnconnected=off
  T_shaft (pu) : Outport  Port=2  VectorParamsAs1DForOutWhenUnconnected=off
  wires:
  wbase/1 -> Discrete-Time Integrator1/1
  Discrete-Time Integrator1/1 -> Stiffness/1
  Stiffness/1 -> Sum2/1
  Sum/1 -> 1_2H_WT/1
  1_2H_WT/1 -> Discrete-Time Integrator/1
  Discrete-Time Integrator/1 -> Sum1/1, W_wt (pu)/1
  Generator speed (pu)/1 -> Sum1/2
  Sum1/1 -> wbase/1, Mutual damping/1
  Mutual damping/1 -> Sum2/2
  Sum2/1 -> Sum/2, T_shaft (pu)/1
  T_wt (pu)/1 -> Sum/1

== system Microgrid_transition_model_092221/../Inverter and DC-DC Converter Average Models ==
  note: Current of the boost converter diode
      | This diode is not illustrated in the average model
  note: Inverter and DC-DC Boost Converter
      | Average Models
  note: DC-DC Converter
      | Average Model
  note: Vab Vbc Inverter
      | Average Model
  note: Pac=Vab*Ia -Vbc*Ic
      | Pdc=Vdc*Idc
  IL : Inport
  Iabc_grid_conv : Inport  Port=2
  Uctrl_inverter : Inport  Port=3
  Duty_Cycle : Inport  Port=4
  0.1 : Gain  Gain=0.5
  0.2 : Gain  Gain=-1
  0.5 : Gain  Gain=0.5
  1/C : Gain  Gain=1/C_DClink
  Constant2 : Constant
  Demux : Demux  Outputs=3
  Demux2 : Demux  Outputs=3
  Discrete-Time Integrator : DiscreteIntegrator  InitialCondition=Vdc_nom  SampleTime=Ts  LimitOutput=on  LowerSaturationLimit=eps  ICPrevOutput=DiscIntNeverNeededParam  ICPrevScaledInput=DiscIntNeverNeededParam
  Product{1..4,6..7} (6 alike) : Product  RndMeth=Zero
  Product5 : Product  Inputs=*/  RndMeth=Zero
  Saturation Dynamic : simulink/Discontinuities/Saturation Dynamic  OutMin=[]  OutMax=[]  OutDataTypeStr=Inherit: Same as second input  OutDataType=sfix(16)  OutScaling=2^-10  DoSatur=off
  Saturation Dynamic1 : simulink/Discontinuities/Saturation Dynamic  OutMin=[]  OutMax=[]  OutDataTypeStr=Inherit: Same as second input  OutDataType=sfix(16)  OutScaling=2^-10  DoSatur=off
  Subtract1 : Sum  Inputs=+-
  Subtract2 : Sum  Inputs=+-
  Subtract3 : Sum  Inputs=+-
  Subtract4 : Sum
  Sum : Sum  Inputs=|+-
  Terminator : Terminator
  pu->A : Gain  Gain=Pnom/(3*sqrt(2)/pi*Vnom_gen)  SaturateOnIntegerOverflow=on  OutDataTypeStr=Inherit: Same as input  ParamDataTypeStr=Inherit: Same as input
  "pu->A " : Gain  Gain=Pnom/sqrt(3)/Vnom*sqrt(2)  SaturateOnIntegerOverflow=on  OutDataTypeStr=Inherit: Same as input  ParamDataTypeStr=Inherit: Same as input
  Vab (V) : Outport  VectorParamsAs1DForOutWhenUnconnected=off
  Vbc (V) : Outport  Port=2  VectorParamsAs1DForOutWhenUnconnected=off
  Vswitch (V) : Outport  Port=3  VectorParamsAs1DForOutWhenUnconnected=off
  Vdc (V) : Outport  Port=4  VectorParamsAs1DForOutWhenUnconnected=off
  wires:
  pu->A/1 -> Product2/2
  [Idiode] -> Subtract4/1  "Idiode"
  Saturation Dynamic1/1 -> [Vbc], Vbc (V)/1
  Saturation Dynamic/1 -> [Vab], Vab (V)/1
  Uctrl_inverter/1 -> Demux2/1
  0.2/1 -> Saturation Dynamic1/3, Saturation Dynamic/3
  0.1/1 -> Saturation Dynamic1/2  "Vbc_avg"
  0.5/1 -> Saturation Dynamic/2  "Vab_avg"
  Demux2/1 -> Subtract3/1
  Demux2/2 -> Subtract1/1, Subtract3/2
  Demux2/3 -> Subtract1/2
  Product6/1 -> 0.5/1
  Product7/1 -> 0.1/1
  Subtract3/1 -> Product6/1
  Subtract1/1 -> Product7/1
  [Vdc] -> Product7/2, Product6/2, Saturation Dynamic/1, Saturation Dynamic1/1, 0.2/1
  Product5/1 -> Subtract4/2  "Idc grid converter"
  [Vbc] -> Product4/1
  [Vab] -> Product3/1
  Demux/3 -> Product4/2  "Ic"
  Subtract2/1 -> Product5/1  "Pac"
  Product3/1 -> Subtract2/1
  Product4/1 -> Subtract2/2
  Duty_Cycle/1 -> Sum/2
  Iabc_grid_conv/1 -> "pu->A "/1
  Demux/2 -> Terminator/1
  "pu->A "/1 -> Demux/1
  Demux/1 -> Product3/2  "Ia"
  Subtract4/1 -> 1/C/1
  Discrete-Time Integrator/1 -> [Vdc], Product5/2, Vdc (V)/1
  1/C/1 -> Discrete-Time Integrator/1
  Constant2/1 -> Sum/1
  Sum/1 -> Product1/2, Product2/1
  IL/1 -> pu->A/1
  [Vdc] -> Product1/1
  Product2/1 -> [Idiode]
  Product1/1 -> Vswitch (V)/1

== system Microgrid_transition_model_092221/../Wind Turbine1 ==
  W_wt (pu) : Inport
  Pitch angle (deg) : Inport  Port=2
  Wind speed (m/s) : Inport  Port=3
  ->pu : Gain  Gain=1/Prated
  2-D Lookup Table1 : Lookup_n-D  BreakpointsForDimension1=breakpoints1  BreakpointsForDimension2=breakpoints2  Table=cp_table_data  InternalRulePriority=Speed  RndMeth=Simplest  InputSameDT=on
  Avoid div. by zero : Saturate  UpperLimit=inf  LowerLimit=eps
  "Avoid div. by zero " : Saturate  UpperLimit=inf  LowerLimit=eps
  Fcn1 : Fcn  Expr=K1*u[2]/u[1]
  Fcn2 : Fcn  Commented=on  Expr=c1*(c6*u[1] + (-c4 - c3*(2.5 + u[2]) + c2*(1/(u[1] + c7*(2.5 + u[2])) -c8/(1 + (2.5 + u[2])^3)))/exp(c5*(1/(u[1] + c7*(2.5 + u[2])) - c8/(1 + (2.5 + u[2])^3))))
  "K2*Cp*wind^3 " : Fcn  Expr=K2*u[1]^3*u[2]
  Mux : Mux  Inputs=2
  Mux2 : Mux  Inputs=2
  Product2 : Product  Inputs=*/  InputSameDT=on  SaturateOnIntegerOverflow=on  OutDataTypeStr=Inherit: Same as first input
  Tt (pu) : Outport  VectorParamsAs1DForOutWhenUnconnected=off
  wires:
  "K2*Cp*wind^3 "/1 -> ->pu/1
  "Avoid div. by zero "/1 -> Product2/2, Mux/2
  Avoid div. by zero/1 -> Mux/1, Mux2/1
  W_wt (pu)/1 -> "Avoid div. by zero "/1
  Pitch angle (deg)/1 -> 2-D Lookup Table1/2
  Mux2/1 -> "K2*Cp*wind^3 "/1
  2-D Lookup Table1/1 -> Mux2/2  "Cp"
  Mux/1 -> Fcn1/1
  Fcn1/1 -> 2-D Lookup Table1/1  "lambda"
  Wind speed (m/s)/1 -> Avoid div. by zero/1
  Product2/1 -> Tt (pu)/1
  ->pu/1 -> Product2/1  "power_pu"

== system Microgrid_transition_model_092221/../Wind Turbine2 ==
  W_wt (pu) : Inport
  Pitch angle (deg) : Inport  Port=2
  Wind speed (m/s) : Inport  Port=3
  ->pu : Gain  Gain=1/Prated
  Avoid div. by zero : Saturate  UpperLimit=inf  LowerLimit=eps
  "Avoid div. by zero " : Saturate  UpperLimit=inf  LowerLimit=eps
  Fcn1 : Fcn  Expr=K1*u[2]/u[1]
  Fcn2 : Fcn  Expr=c1*(c6*u[1] + (-c4 - c3*(2.5 + u[2]) + c2*(1/(u[1] + c7*(2.5 + u[2])) -c8/(1 + (2.5 + u[2])^3)))/exp(c5*(1/(u[1] + c7*(2.5 + u[2])) - c8/(1 + (2.5 + u[2])^3))))
  "K2*Cp*wind^3 " : Fcn  Expr=K2*u[1]^3*u[2]
  Mux : Mux  Inputs=2
  Mux1 : Mux  Inputs=2
  Mux2 : Mux  Inputs=2
  Product2 : Product  Inputs=*/  InputSameDT=on  SaturateOnIntegerOverflow=on  OutDataTypeStr=Inherit: Same as first input
  Tt (pu) : Outport  VectorParamsAs1DForOutWhenUnconnected=off
  wires:
  ->pu/1 -> Product2/1  "power_pu"
  Product2/1 -> Tt (pu)/1
  Wind speed (m/s)/1 -> Avoid div. by zero/1
  Fcn1/1 -> Mux1/1  "lambda"
  Mux1/1 -> Fcn2/1
  Mux/1 -> Fcn1/1
  Fcn2/1 -> Mux2/2  "Cp"
  Mux2/1 -> "K2*Cp*wind^3 "/1
  Pitch angle (deg)/1 -> Mux1/2
  W_wt (pu)/1 -> "Avoid div. by zero "/1
  Avoid div. by zero/1 -> Mux2/1, Mux/1
  "Avoid div. by zero "/1 -> Mux/2, Product2/2
  "K2*Cp*wind^3 "/1 -> ->pu/1
